simulink model "SiMappedEngineV"  (R2024b)
settings: Solver=FixedStepAuto  StartTime=0.0  StopTime=inf  FixedStep=0.001  RelTol=1e-3  EnableMultiTasking=on
model workspace (MAT data in the model file):
  AccPwrbp = [0 3.07795609935]
  AccSpdbp = [256.496417196 641.24104299]
  AfrStoich = 14.6
  Cps = 2
  NCyl = 6
  Pstd = 101325
  Rair = 287
  Tstd = 293.15
  Vd = 0.00359999893917
  f_air = [0 0 0 0 0 0 0 0 0 0 0 0 ... (256 elements, 16x16)]
  f_co = [0 0 0 0 0 0 0 0 0 0 0 0 ... (256 elements, 16x16)]
  f_co2 = [0 0 0 0 0 0 0 0 0 0 0 0 ... (256 elements, 16x16)]
  f_eff = [0 350.753466782 328.05948506 313.268671005 303.348195903 297.340325295 293.478152627 291.797966365 291.798018438 291.798071207 291.798124411 291.798172385 ... (256 elements, 16x16)]
  f_fuel = [0 0 0 0 0 0 0 0 0 0 0 0 ... (256 elements, 16x16)]
  f_hc = [0 0 0 0 0 0 0 0 0 0 0 0 ... (256 elements, 16x16)]
  f_nox = [0 0 0 0 0 0 0 0 0 0 0 0 ... (256 elements, 16x16)]
  f_pm = [0 0 0 0 0 0 0 0 0 0 0 0 ... (256 elements, 16x16)]
  f_tbrake = [0 80.7204067348 99.7652469493 118.69381236 137.622341282 156.550901814 175.479464551 180.804356543 180.803988299 180.803666493 180.803369276 180.803064185 ... (256 elements, 16x16)]
  f_tbrake_n_bpt = [0 641.24104299 900.790988962 1160.34093493 1419.89088091 1679.44082688 1938.99077285 2198.54071882 2458.09066479 2717.64061077 2977.19055674 3236.74050271 ... (16 elements, 1x16)]
  f_tbrake_t_bpt = [0 35 53.9285714286 72.8571428571 91.7857142857 110.714285714 129.642857143 148.571428571 167.5 186.428571429 205.357142857 224.285714286 ... (16 elements, 1x16)]
  f_texh = [762.273993769 762.941951792 776.57840337 790.535834434 800.856847168 863.73255561 896.950654556 906.72093477 906.720129025 906.720506327 906.719870748 906.718704777 ... (256 elements, 16x16)]
libraries: autolibutils x2, autolibsharedmappedengines x1
(part 2 of 2)

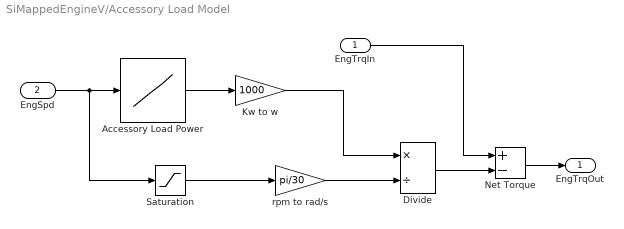
== system SiMappedEngineV/Accessory Load Model ==
  EngTrqIn : Inport
  EngSpd : Inport  Port=2
  Accessory Load Power : Lookup_n-D  NumberOfTableDimensions=1  LookupTableObject=''  BreakpointsForDimension1=AccSpdbp  Table=AccPwrbp  ExtrapMethod=Clip  InternalRulePriority=Speed  RndMeth=Simplest
  Divide : Product  Inputs=*/
  Kw to w : Gain  Gain=1000
  Net Torque : Sum  Inputs=+-
  Saturation : Saturate  UpperLimit=Inf  LowerLimit=300
  rpm to rad/s : Gain  Gain=pi/30
  EngTrqOut : Outport  Unit=N*m  VectorParamsAs1DForOutWhenUnconnected=off
  wires:
  Divide/1 -> Net Torque/2
  Accessory Load Power/1 -> Kw to w/1
  EngSpd/1 -> Saturation/1, Accessory Load Power/1
  Saturation/1 -> rpm to rad/s/1
  rpm to rad/s/1 -> Divide/2
  Net Torque/1 -> EngTrqOut/1
  Kw to w/1 -> Divide/1
  EngTrqIn/1 -> Net Torque/1
